simulink model "bloque_b_completoemi"  (Simulink 5.0)
settings: Solver=ode45  StartTime=0.0  StopTime=25.0  RelTol=1e-3
undefined symbols (not defined in the file): a, d, k1, k2, q, Vd, Vm
libraries: dspsigops x1
settings Model: LastModifiedBy=pc1

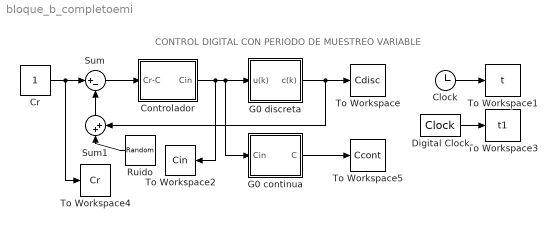
== system bloque_b_completoemi ==
  note: CONTROL DIGITAL CON PERIODO DE MUESTREO VARIABLE
  Clock : Clock
      settings: Decimation=10
  Controlador : Subsystem
  Cr : Constant
  Digital Clock : DigitalClock  SampleTime=0.01
  G0 continua : Subsystem
  G0 discreta : Subsystem
  Ruido : RandomNumber  Orientation=left  Variance=0.01  Seed=5  SampleTime=0.1
  Sum : Sum  Inputs=|+-  SaturateOnIntegerOverflow=on
  Sum1 : Sum  Orientation=up  Inputs=|++  SaturateOnIntegerOverflow=on
  To Workspace : ToWorkspace  VariableName=Cdisc  SampleTime=0.01  SaveFormat=Array
  To Workspace1 : ToWorkspace  VariableName=t  SampleTime=-1  SaveFormat=Array
  To Workspace2 : ToWorkspace  VariableName=Cin  SampleTime=0.01  SaveFormat=Array
  To Workspace3 : ToWorkspace  VariableName=t1  SampleTime=0.01  SaveFormat=Array
  To Workspace4 : ToWorkspace  VariableName=Cr  SampleTime=0.01  SaveFormat=Array
  To Workspace5 : ToWorkspace  VariableName=Ccont  SampleTime=-1  SaveFormat=Array
  wires:
  Controlador/1(Cin) -> To Workspace2/1, G0 discreta/1(u(k)), G0 continua/1(Cin)
  G0 discreta/1(c(k)) -> To Workspace/1, Sum1/2
  Cr/1 -> Sum/1, To Workspace4/1
  Sum/1 -> Controlador/1(Cr-C)
  Clock/1 -> To Workspace1/1
  Digital Clock/1 -> To Workspace3/1
  G0 continua/1(C) -> To Workspace5/1
  Sum1/1 -> Sum/2
  Ruido/1 -> Sum1/1

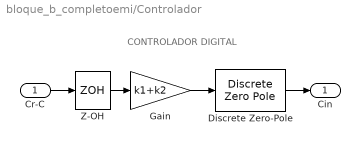
== system bloque_b_completoemi/Controlador ==
  note: CONTROLADOR DIGITAL
  Cr-C : Inport
  Discrete Zero-Pole : DiscreteZeroPole  Zeros=[2/3]  Poles=[1]  Gain=1  SampleTime=Vd/(d*q)
  Gain : Gain  Gain=k1+k2  SaturateOnIntegerOverflow=on
  Z-OH : ZeroOrderHold  SampleTime=Vd/(d*q)
  Cin : Outport
  wires:
  Gain/1 -> Discrete Zero-Pole/1
  Z-OH/1 -> Gain/1
  Discrete Zero-Pole/1 -> Cin/1
  Cr-C/1 -> Z-OH/1

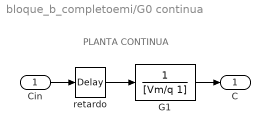
== system bloque_b_completoemi/G0 continua ==
  note: PLANTA CONTINUA
  Cin : Inport
  G1 : TransferFcn  Denominator=[Vm/q 1]
  retardo : TransportDelay  DelayTime=Vd/q
  C : Outport
  wires:
  retardo/1 -> G1/1
  G1/1 -> C/1
  Cin/1 -> retardo/1

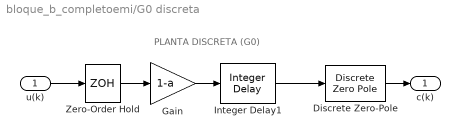
== system bloque_b_completoemi/G0 discreta ==
  note: PLANTA DISCRETA (G0)
  u(k) : Inport
  Discrete Zero-Pole : DiscreteZeroPole  Zeros=[0]  Poles=[a]  Gain=1  SampleTime=Vd/(q*d)
  Gain : Gain  Gain=1-a  SaturateOnIntegerOverflow=on
  Integer Delay1 : dspsigops/Integer Delay  delay=d+1  ic=0  reset_popup=None
  Zero-Order Hold : ZeroOrderHold  SampleTime=Vd/(d*q)
  c(k) : Outport
  wires:
  Zero-Order Hold/1 -> Gain/1
  Gain/1 -> Integer Delay1/1
  Integer Delay1/1 -> Discrete Zero-Pole/1
  Discrete Zero-Pole/1 -> c(k)/1
  u(k)/1 -> Zero-Order Hold/1
